simulink model "untitlednew"  (Simulink 8.0)
settings: Solver=ode3  StartTime=0.0  StopTime=stop_time  FixedStep=step_time  MaxStep=step_time  MinStep=step_time  RelTol=1e-3
values from neighbouring files (symbols this model uses):
  Exp_Lamda = 7.9    [main_1.m]
  mean_wind = 15    [main_1.m]
  R = 38.5    [main_1.m]    (also in test.m)
settings Model: Creator=dujiexian  LastModifiedBy=Administrator

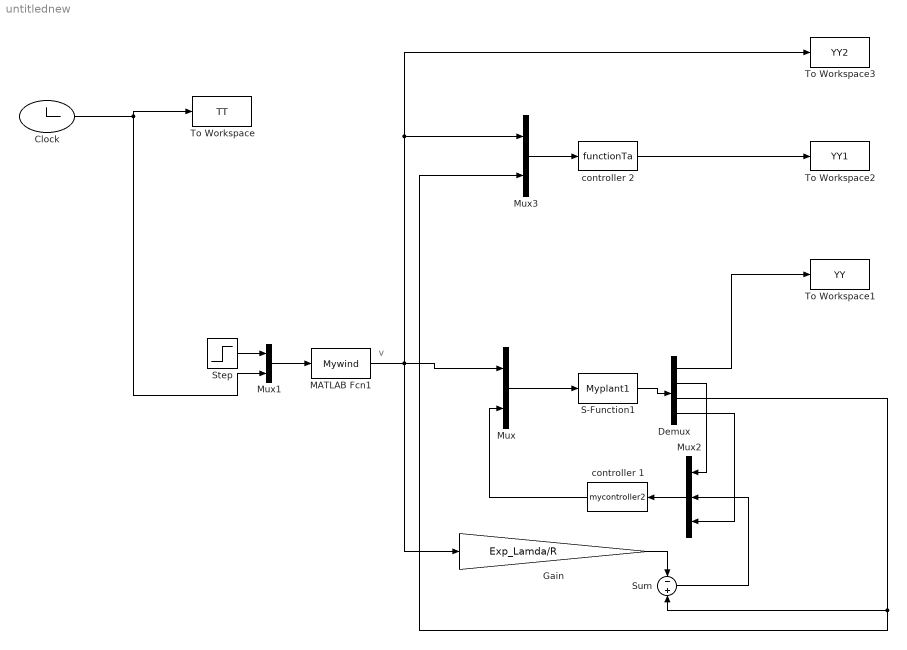
== system untitlednew ==
  note: v
  Clock : Clock
  Demux : Demux
  Gain : Gain  Gain=Exp_Lamda/R
  MATLAB Fcn1 : MATLABFcn  MATLABFcn=Mywind
  Mux : Mux  Inputs=2
  Mux1 : Mux  Inputs=2
  Mux2 : Mux  Inputs=3
  Mux3 : Mux  Inputs=2
  S-Function1 : S-Function  FunctionName=Myplant1  EnableBusSupport=off
  Step : Step  Time=0  After=mean_wind  SampleTime=0
  Sum : Sum  Inputs=-+
  To Workspace : ToWorkspace  VariableName=TT  SampleTime=-1
  To Workspace1 : ToWorkspace  VariableName=YY  SampleTime=-1
  To Workspace2 : ToWorkspace  VariableName=YY1  SampleTime=-1
  To Workspace3 : ToWorkspace  VariableName=YY2  SampleTime=-1
  controller 1 : MATLABFcn  MATLABFcn=mycontroller2
  controller 2 : MATLABFcn  MATLABFcn=functionTa
  wires:
  Clock/1 -> To Workspace/1, Mux1/2
  MATLAB Fcn1/1 -> Gain/1, To Workspace3/1, Mux3/1, Mux/1
  Step/1 -> Mux1/1
  Mux1/1 -> MATLAB Fcn1/1
  Mux/1 -> S-Function1/1
  Demux/1 -> To Workspace1/1
  S-Function1/1 -> Demux/1
  Demux/2 -> Mux2/1
  Demux/4 -> Mux2/3
  Mux2/1 -> controller 1/1
  controller 1/1 -> Mux/2
  Demux/3 -> Mux3/2, Sum/2
  Sum/1 -> Mux2/2
  Mux3/1 -> controller 2/1
  controller 2/1 -> To Workspace2/1
  Gain/1 -> Sum/1
